simulink model "experiment_1"  (R2023b)
settings: Solver=VariableStepAuto  StartTime=0.0  StopTime=300  RelTol=1e-3
undefined symbols (not defined in the file or in its folder): den_phi, den_theta, g0, Ip, Ir, Lp, Lr, mp, mr, num_phi, num_theta, param, rot_pend
libraries: simulink_extras x3
settings Model: Creator=Mark  LastModifiedBy=Mark
settings DataIOCC: InitialState=x0

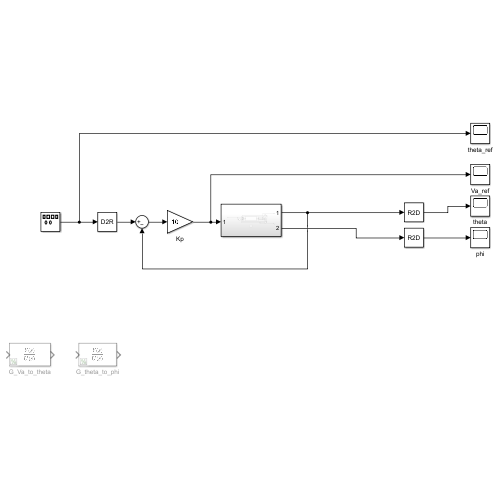
[thumbnail: Simulink's stored preview of the top-level diagram]
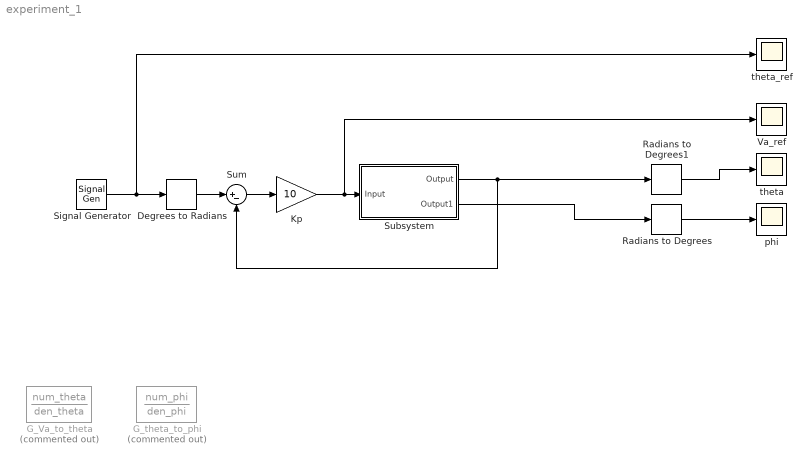
== system experiment_1 ==
  Degrees to Radians : simulink_extras/Transformations/Degrees to Radians
  G_Va_to_theta : TransferFcn  Commented=on  Numerator=num_theta  Denominator=den_theta
  G_theta_to_phi : TransferFcn  Commented=on  Numerator=num_phi  Denominator=den_phi
  Kp : Gain  Gain=10
  Radians to Degrees : simulink_extras/Transformations/Radians to Degrees
  Radians to Degrees1 : simulink_extras/Transformations/Radians to Degrees
  Signal Generator : SignalGenerator  WaveForm=square  Amplitude=20  Frequency=0.05
  Subsystem : Subsystem
  Sum : Sum  Inputs=|+-
  Va_ref : Scope
  phi : Scope
  theta : Scope
  theta_ref : Scope
  wires:
  Kp/1 -> Va_ref/1, Subsystem/1(Input)
  Subsystem/2(Output1) -> Radians to Degrees/1
  Sum/1 -> Kp/1
  Degrees to Radians/1 -> Sum/1
  Radians to Degrees/1 -> phi/1
  Radians to Degrees1/1 -> theta/1
  Subsystem/1(Output) -> Radians to Degrees1/1, Sum/2
  Signal Generator/1 -> theta_ref/1, Degrees to Radians/1

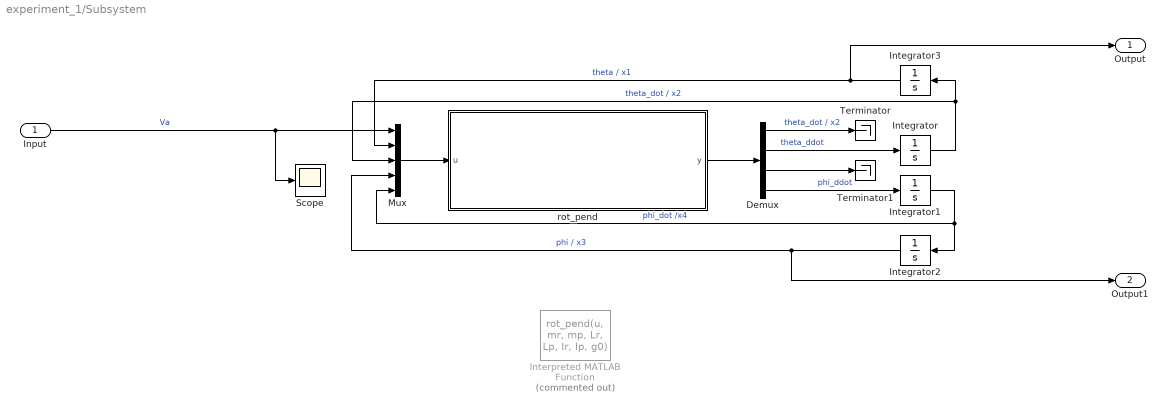
== system experiment_1/Subsystem ==
  Input : Inport
  Demux : Demux
  Integrator{,1..3} (4 alike) : Integrator
  Interpreted MATLAB Function : MATLABFcn  Commented=on  MATLABFcn=rot_pend(u, mr, mp, Lr, Lp, Ir, Ip, g0)  OutputDimensions=4  OutputSignalType=real
  Mux : Mux  Inputs=5
  Scope : Scope
  Terminator : Terminator
  Terminator1 : Terminator
  rot_pend : Subsystem
  Output : Outport
  Output1 : Outport  Port=2
  wires:
  Input/1 -> Scope/1, Mux/1  "Va"
  Integrator2/1 -> Output1/1, Mux/4  "phi / x3"
  Integrator/1 -> Integrator3/1, Mux/3  "theta_dot / x2"
  Mux/1 -> rot_pend/1(u)
  rot_pend/1(y) -> Demux/1
  Integrator1/1 -> Mux/5, Integrator2/1  "phi_dot /x4"
  Integrator3/1 -> Mux/2, Output/1  "theta / x1"
  Demux/4 -> Integrator1/1  "phi_ddot"
  Demux/2 -> Integrator/1  "theta_ddot"
  Demux/1 -> Terminator/1  "theta_dot / x2"
  Demux/3 -> Terminator1/1

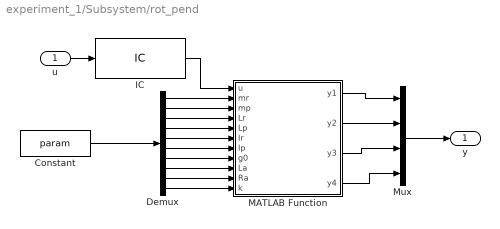
== system experiment_1/Subsystem/rot_pend ==
  u : Inport
  Constant : Constant  Value=param  VectorParams1D=off
  Demux : Demux  Outputs=10
  IC : InitialCondition  Value=[0 0 0 pi 0]'
  MATLAB Function : MATLAB Function  TreatAsAtomicUnit=on
  Mux : Mux
  y : Outport
  wires:
  Demux/3 -> MATLAB Function/4(Lr)
  Demux/5 -> MATLAB Function/6(Ir)
  Demux/4 -> MATLAB Function/5(Lp)
  Demux/7 -> MATLAB Function/8(g0)
  Demux/2 -> MATLAB Function/3(mp)
  Demux/6 -> MATLAB Function/7(Ip)
  Demux/1 -> MATLAB Function/2(mr)
  IC/1 -> MATLAB Function/1(u)
  Constant/1 -> Demux/1
  MATLAB Function/1(y1) -> Mux/1
  MATLAB Function/2(y2) -> Mux/2
  MATLAB Function/3(y3) -> Mux/3
  MATLAB Function/4(y4) -> Mux/4
  Mux/1 -> y/1
  Demux/8 -> MATLAB Function/9(La)
  Demux/9 -> MATLAB Function/10(Ra)
  Demux/10 -> MATLAB Function/11(k)
  u/1 -> IC/1

== matlab function experiment_1/Subsystem/rot_pend/MATLAB Function ==
  data: u input; y1 output; mr input; mp input; Lr input; Lp input; Ir input; Ip input; g0 input; La input; Ra input; y2 output; y3 output; y4 output; k input
function [y1,y2,y3,y4] = rot_pend(u, mr, mp, Lr, Lp, Ir, Ip, g0,La, Ra, k)
%UNTITLED Summary of this function goes here
%   Detailed explanation goes here
% u(1) = Va
x1 = u(2) ; % theta
x2 = u(3) ; % theta_dot
x3 = u(4) ; % phi
x4 = u(5) ; % phi_dot

H = [(mp*(Lr^2+(Lp^2*(sin(x3))^2)))+4.7912e-05           mp*Lr*Lp*cos(x3);
                     mp*Lr*Lp*cos(x3)                              (mp*Lp^2)+Ip] ;

Q = [mp*Lp^2*sin(x3)*cos(x3)*x4                     (mp*Lp^2*sin(x3)*cos(x3)*x2)-(mp*Lr*Lp*sin(x3)*x4);
     -mp*Lp^2*sin(x3)*cos(x3)*x4                                                   0                                   ] ;

g = [           0     ;
     -mp*g0*Lp*sin(x3)] ;
tau = [((k/Ra)*u(1))-((k^2/Ra)*x2);
                    0                   ] ;

q_ddot = H\[tau - Q*[x2 x4]' - g] ;


y1 = x2 ;
y2 = q_ddot(1) ;
y3 = x4 ;
y4 = q_ddot(2) ;


%Ir+mr*(Lr/2)^2)
